simulink model "KR6_JacobianValidation"  (R2018a)
settings: Solver=VariableStepAuto  StartTime=0.0  StopTime=inf  FixedStep=1e-6  RelTol=1e-3
libraries: vrlib x8, simulink x7, KR6_Lib x1, dspindex x1
settings Model: Creator=Pedro Ramalho  LastModifiedBy=Pedro Ramalho

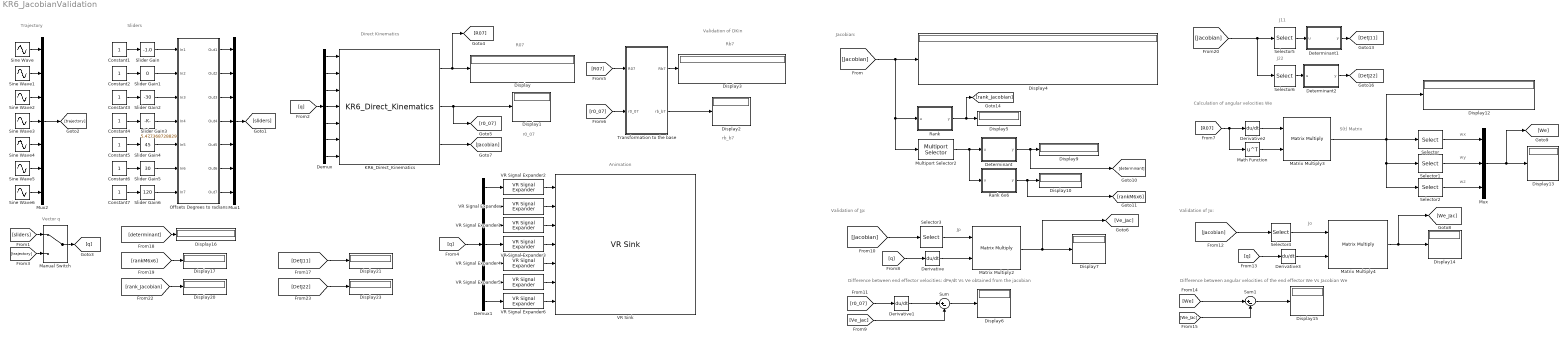
== system KR6_JacobianValidation ==
  note: S(t) Matrix
  note: Vector q
  note: Sliders
  note: Trajectory
  note: Animation
  note: Direct Kinematics
  note: R07
  note: r0_07
  note: Rb7
  note: rb_b7
  note: Validation of DKin
  note: Validation of Jp:
  note: Difference between end effector velocities: dPe/dt Vs Ve obtained from the jacobian
  note: Jp
  note: Jacobian:
  note: Validation of Jo:
  note: Jo
  note: Difference between angular velocities of the end effector We Vs Jacobian We
  note: wx
  note: wy
  note: wz
  note: Calculation of angular velocities We
  note: J22
  note: J11
  " Determinant" : MATLAB Function  TreatAsAtomicUnit=on
  " Determinant1" : MATLAB Function  TreatAsAtomicUnit=on
  " Determinant2" : MATLAB Function  TreatAsAtomicUnit=on
  Constant{1..7} (7 alike) : Constant
  Demux : Demux  Outputs=7
  Demux1 : Demux  Outputs=7
  Derivative{,1..3} (4 alike) : Derivative
  Display{,1..7,9..10,12..17,20..21,23} (19 alike) : Display
      Display settings: Decimation=2
  KR6_Direct_Kinematics : KR6_Lib/KR6_Direct_Kinematics
  Manual Switch : ManualSwitch
  Math Function : Math  Operator=transpose  SaturateOnIntegerOverflow=on
  Matrix Multiply2 : Product  Multiplication=Matrix(*)
  Matrix Multiply3 : Product  Multiplication=Matrix(*)
  Matrix Multiply4 : Product  Multiplication=Matrix(*)
  Multiport Selector2 : dspindex/Multiport Selector  rowsOrCols=Columns  idxCellArray={[2:7]}  idxErrMode=Clip Index
  Mux : Mux  Inputs=3
  Mux1 : Mux  Inputs=7
  Mux2 : Mux  Inputs=7
  Offsets Degrees to radians : Subsystem
  Rank : MATLAB Function  TreatAsAtomicUnit=on
  Rank 6x6 : MATLAB Function  TreatAsAtomicUnit=on
  Selector : Selector  NumberOfDimensions=2  InputPortWidth=3  IndexOptions=Index vector (dialog),Index vector (dialog)  Indices=[3],[2]  OutputSizes=1,1
  Selector1 : Selector  NumberOfDimensions=2  InputPortWidth=3  IndexOptions=Index vector (dialog),Index vector (dialog)  Indices=[1],[3]  OutputSizes=1,1
  Selector2 : Selector  NumberOfDimensions=2  InputPortWidth=3  IndexOptions=Index vector (dialog),Index vector (dialog)  Indices=[2],[1]  OutputSizes=1,1
  Selector3 : Selector  NumberOfDimensions=2  InputPortWidth=3  IndexOptions=Index vector (dialog),Index vector (dialog)  Indices=1:3,1:7  OutputSizes=1,1
  Selector4 : Selector  NumberOfDimensions=2  InputPortWidth=3  IndexOptions=Index vector (dialog),Index vector (dialog)  Indices=4:6,1:7  OutputSizes=1,1
  Selector5 : Selector  NumberOfDimensions=2  InputPortWidth=3  IndexOptions=Index vector (dialog),Index vector (dialog)  Indices=1:3,2:4  OutputSizes=1,1
  Selector6 : Selector  NumberOfDimensions=2  InputPortWidth=3  IndexOptions=Index vector (dialog),Index vector (dialog)  Indices=4:6,5:7  OutputSizes=1,1
  Sine Wave : Sin  Frequency=0.5  SampleTime=0
  Sine Wave1 : Sin  Amplitude=3  Frequency=0.5  SampleTime=0
  Sine Wave2 : Sin  Bias=-1.5  Frequency=0.5  SampleTime=0
  Sine Wave3 : Sin  Amplitude=0.5  Frequency=0.5  SampleTime=0
  Sine Wave4 : Sin  Frequency=0.5  SampleTime=0
  Sine Wave5 : Sin  Amplitude=1.5  Frequency=0.5  SampleTime=0
  Sine Wave6 : Sin  Amplitude=1.5  Frequency=0.5  SampleTime=0
  Slider Gain : simulink/Math Operations/Slider Gain  gain=-1.0  low=-1  high=1
  Slider Gain1 : simulink/Math Operations/Slider Gain  gain=0  low=-180  high=180
  Slider Gain2 : simulink/Math Operations/Slider Gain  gain=-30  low=-180  high=180
  Slider Gain3 : simulink/Math Operations/Slider Gain  gain=5.477368728829  low=-180  high=180
  Slider Gain4 : simulink/Math Operations/Slider Gain  gain=45  low=-180  high=180
  Slider Gain5 : simulink/Math Operations/Slider Gain  gain=30  low=-180  high=180
  Slider Gain6 : simulink/Math Operations/Slider Gain  gain=120  low=-180  high=180
  Sum : Sum  Inputs=|+-
  Sum1 : Sum  Inputs=|+-
  Transformation to the base : Subsystem
  VR Signal Expander{,1,3..6} (6 alike) : vrlib/VR Signal Expander  outwidth=4  outidx=4
      settings: SourceProductName=Simulink 3D Animation  SourceProductBaseCode=VR
  VR Signal Expander2 : vrlib/VR Signal Expander  outwidth=3  outidx=3
      settings: SourceProductName=Simulink 3D Animation  SourceProductBaseCode=VR
  VR Sink : vrlib/VR Sink  InstantiateOnLoad=on  SampleTime=0.1  ViewEnable=on  RemoteChange=off  RemoteView=off  FieldsWritten=Jt1_DH_dv.translation.3.1.1.double#Jt2_DH_dv.rotation.4.1.1.double#Jt3_DH_dv.rotation.4.1.1.double#Jt4_DH_dv.rotation.4.1.1.double#Jt5_DH_dv.rotation.4.1.1.double#Jt6_DH_dv.rotation.4.1.1.double#Jt7_DH_dv.rotation.4.1.1.double  WorldFileName=vrrobotKR6.wrl  WorldDescription=D-H Reference Frames for Virtual Reality Robot  AutoView=off  VideoDimensions=[]  AllowVariableSize=off
      settings: SourceProductBaseCode=VR
  wires:
  KR6_Direct_Kinematics/1 -> [R07], Display/1
  KR6_Direct_Kinematics/2 -> [r0_07], Display1/1
  Constant1/1 -> Slider Gain/1
  Constant2/1 -> Slider Gain1/1
  Constant3/1 -> Slider Gain2/1
  Constant4/1 -> Slider Gain3/1
  Constant5/1 -> Slider Gain4/1
  Constant6/1 -> Slider Gain5/1
  Constant7/1 -> Slider Gain6/1
  Sine Wave/1 -> Mux2/1
  Slider Gain/1 -> Offsets Degrees to radians/1(In1)
  Slider Gain1/1 -> Offsets Degrees to radians/2(In2)
  Slider Gain2/1 -> Offsets Degrees to radians/3(In3)
  Slider Gain3/1 -> Offsets Degrees to radians/4(In4)
  Slider Gain4/1 -> Offsets Degrees to radians/5(In5)
  Slider Gain5/1 -> Offsets Degrees to radians/6(In6)
  Slider Gain6/1 -> Offsets Degrees to radians/7(In7)
  Offsets Degrees to radians/1(Out1) -> Mux1/1
  Offsets Degrees to radians/2(Out2) -> Mux1/2
  Offsets Degrees to radians/3(Out3) -> Mux1/3
  Offsets Degrees to radians/4(Out4) -> Mux1/4
  Offsets Degrees to radians/5(Out5) -> Mux1/5
  Offsets Degrees to radians/6(Out6) -> Mux1/6
  Offsets Degrees to radians/7(Out7) -> Mux1/7
  [sliders] -> Manual Switch/1
  [trajectory] -> Manual Switch/2
  Mux1/1 -> [sliders]
  Demux/1 -> KR6_Direct_Kinematics/1
  Demux/2 -> KR6_Direct_Kinematics/2
  Demux/3 -> KR6_Direct_Kinematics/3
  Demux/4 -> KR6_Direct_Kinematics/4
  Demux/5 -> KR6_Direct_Kinematics/5
  Demux/6 -> KR6_Direct_Kinematics/6
  Demux/7 -> KR6_Direct_Kinematics/7
  [q] -> Demux/1
  [q] -> Demux1/1
  Demux1/1 -> VR Signal Expander2/1
  Demux1/3 -> VR Signal Expander1/1
  Demux1/6 -> VR Signal Expander5/1
  Demux1/2 -> VR Signal Expander/1
  Demux1/5 -> VR Signal Expander4/1
  Demux1/4 -> VR Signal Expander3/1
  Demux1/7 -> VR Signal Expander6/1
  Manual Switch/1 -> [q]
  Sine Wave1/1 -> Mux2/2
  Sine Wave2/1 -> Mux2/3
  Sine Wave3/1 -> Mux2/4
  Sine Wave4/1 -> Mux2/5
  Sine Wave5/1 -> Mux2/6
  Sine Wave6/1 -> Mux2/7
  Mux2/1 -> [trajectory]
  Selector3/1 -> Matrix Multiply2/1
  Derivative/1 -> Matrix Multiply2/2
  Sum/1 -> Display6/1
  [r0_07] -> Derivative1/1
  Rank/1(y) -> [rank_Jacobian], Display5/1
  Derivative1/1 -> Sum/1
  Matrix Multiply2/1 -> [Ve_Jac], Display7/1
  [q] -> Derivative/1
  [Jacobian] -> Selector3/1
  [Ve_Jac] -> Sum/2
  [Jacobian] -> Multiport Selector2/1, Rank/1(u), Display4/1
  KR6_Direct_Kinematics/3 -> [Jacobian]
  " Determinant"/1(y) -> [determinant], Display9/1
  Multiport Selector2/1 -> Rank 6x6/1(u), " Determinant"/1(u)
  Rank 6x6/1(y) -> [rankM6x6], Display10/1
  [R07] -> Math Function/1, Derivative2/1
  Derivative2/1 -> Matrix Multiply3/1
  Matrix Multiply3/1 -> Selector2/1, Selector1/1, Selector/1, Display12/1
  Math Function/1 -> Matrix Multiply3/2
  Selector2/1 -> Mux/3
  Selector1/1 -> Mux/2
  Selector/1 -> Mux/1
  Mux/1 -> [We], Display13/1
  [q] -> Derivative3/1
  [Jacobian] -> Selector4/1
  Derivative3/1 -> Matrix Multiply4/2
  Matrix Multiply4/1 -> [We_Jac], Display14/1
  Selector4/1 -> Matrix Multiply4/1
  [We] -> Sum1/1
  [We_Jac] -> Sum1/2
  Sum1/1 -> Display15/1
  VR Signal Expander2/1 -> VR Sink/1
  VR Signal Expander/1 -> VR Sink/2
  VR Signal Expander1/1 -> VR Sink/3
  VR Signal Expander3/1 -> VR Sink/4
  VR Signal Expander4/1 -> VR Sink/5
  VR Signal Expander5/1 -> VR Sink/6
  VR Signal Expander6/1 -> VR Sink/7
  [determinant] -> Display16/1
  [rankM6x6] -> Display17/1
  [rank_Jacobian] -> Display20/1
  [R07] -> Transformation to the base/1(R07)
  [r0_07] -> Transformation to the base/2(r0_07)
  Transformation to the base/1(Rb7) -> Display3/1
  Transformation to the base/2(rb_b7) -> Display2/1
  [DetJ22] -> Display23/1
  [DetJ11] -> Display21/1
  Selector5/1 -> " Determinant1"/1(u)
  Selector6/1 -> " Determinant2"/1(u)
  [Jacobian] -> Selector6/1, Selector5/1
  " Determinant1"/1(y) -> [DetJ11]
  " Determinant2"/1(y) -> [DetJ22]

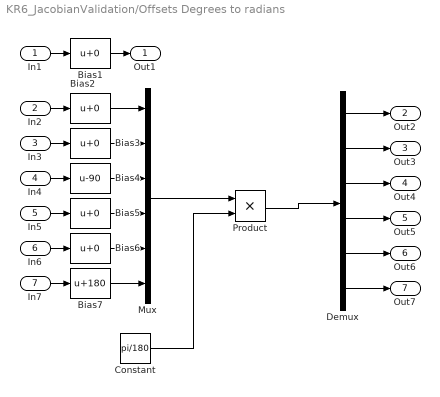
== system KR6_JacobianValidation/Offsets Degrees to radians ==
  In1 : Inport
  In2 : Inport  Port=2
  In3 : Inport  Port=3
  In4 : Inport  Port=4
  In5 : Inport  Port=5
  In6 : Inport  Port=6
  In7 : Inport  Port=7
  Bias{1..3,5..6} (5 alike) : Bias
  Bias4 : Bias  Bias=-90
  Bias7 : Bias  Bias=180
  Constant : Constant  Value=pi/180
  Demux : Demux  Outputs=6
  Mux : Mux  Inputs=6
  Product : Product
  Out1 : Outport
  Out2 : Outport  Port=2
  Out3 : Outport  Port=3
  Out4 : Outport  Port=4
  Out5 : Outport  Port=5
  Out6 : Outport  Port=6
  Out7 : Outport  Port=7
  wires:
  In6/1 -> Bias6/1
  In5/1 -> Bias5/1
  In3/1 -> Bias3/1
  In1/1 -> Bias1/1
  Bias1/1 -> Out1/1
  In7/1 -> Bias7/1
  In4/1 -> Bias4/1
  In2/1 -> Bias2/1
  Bias7/1 -> Mux/6
  Bias2/1 -> Mux/1
  Bias3/1 -> Mux/2
  Bias4/1 -> Mux/3
  Bias5/1 -> Mux/4
  Bias6/1 -> Mux/5
  Mux/1 -> Product/1
  Constant/1 -> Product/2
  Demux/1 -> Out2/1
  Demux/2 -> Out3/1
  Demux/3 -> Out4/1
  Demux/4 -> Out5/1
  Demux/5 -> Out6/1
  Demux/6 -> Out7/1
  Product/1 -> Demux/1

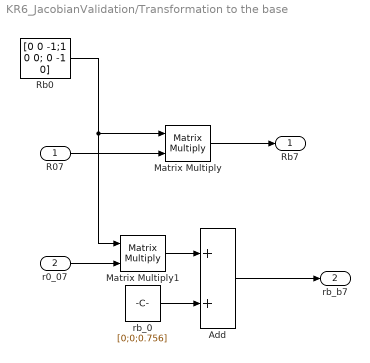
== system KR6_JacobianValidation/Transformation to the base ==
  R07 : Inport
  r0_07 : Inport  Port=2
  Add : Sum
  Matrix Multiply : Product  Multiplication=Matrix(*)
  Matrix Multiply1 : Product  Multiplication=Matrix(*)
  Rb0 : Constant  Value=[0 0 -1;1 0 0; 0 -1 0]
  rb_0 : Constant  Value=[0;0;0.756]
  Rb7 : Outport
  rb_b7 : Outport  Port=2
  wires:
  Matrix Multiply1/1 -> Add/1
  R07/1 -> Matrix Multiply/2
  rb_0/1 -> Add/2
  Rb0/1 -> Matrix Multiply1/1, Matrix Multiply/1
  Matrix Multiply/1 -> Rb7/1
  r0_07/1 -> Matrix Multiply1/2
  Add/1 -> rb_b7/1

== matlab function KR6_JacobianValidation/ Determinant ==
  data: u input; y output
function y = fcn(u)

y = det(u);
%determinante do jacobiano

== matlab function KR6_JacobianValidation/Rank ==
  data: u input; y output
function y = fcn(u)

y = rank(u);
%rank do jacobiano

== matlab function KR6_JacobianValidation/Rank 6x6 ==
  data: u input; y output
function y = fcn(u)

y = rank(u);
%rank do jacobiano

== matlab function KR6_JacobianValidation/ Determinant1 ==
  data: u input; y output
function y = fcn(u)

y = det(u);
%determinante do jacobiano

== matlab function KR6_JacobianValidation/ Determinant2 ==
  data: u input; y output
function y = fcn(u)

y = det(u);
%determinante do jacobiano
